simulink model "subfiltsimplements"  (R2015b)
settings: Solver=FixedStepDiscrete  StartTime=0.0  StopTime=10.0  FixedStep=1  RelTol=1e-3
libraries: Sedea_Sul_filterlib x3
settings Model: Creator=sedur  LastModifiedBy=sedur
settings DataIOCC: SaveFormat=Structure

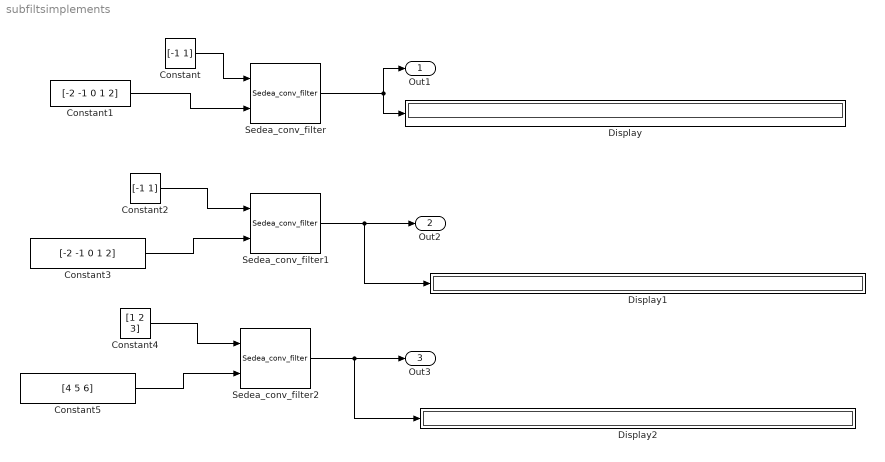
== system subfiltsimplements ==
  Constant : Constant  Value=[-1 1]
  Constant1 : Constant  Value=[-2 -1 0 1 2]
  Constant2 : Constant  Value=[-1 1]
  Constant3 : Constant  Value=[-2 -1 0 1 2]
  Constant4 : Constant  Value=[1 2 3]
  Constant5 : Constant  Value=[4 5 6]
  Display : Display
  Display1 : Display
  Display2 : Display
  Sedea_conv_filter : Sedea_Sul_filterlib/Sedea_conv_filter  shape=full
  Sedea_conv_filter1 : Sedea_Sul_filterlib/Sedea_conv_filter  shape=same
  Sedea_conv_filter2 : Sedea_Sul_filterlib/Sedea_conv_filter  shape=same
  Out1 : Outport
  Out2 : Outport  Port=2
  Out3 : Outport  Port=3
  wires:
  Constant3/1 -> Sedea_conv_filter1/2
  Constant2/1 -> Sedea_conv_filter1/1
  Constant1/1 -> Sedea_conv_filter/2
  Constant/1 -> Sedea_conv_filter/1
  Sedea_conv_filter/1 -> Out1/1, Display/1
  Sedea_conv_filter1/1 -> Display1/1, Out2/1
  Constant5/1 -> Sedea_conv_filter2/2
  Constant4/1 -> Sedea_conv_filter2/1
  Sedea_conv_filter2/1 -> Display2/1, Out3/1
